simulink model "ex2_s"  (Simulink 7.9)
settings: Solver=ode45  StartTime=0.0  StopTime=10.0  RelTol=1e-3
undefined symbols (not defined in the file or in its folder): b1, den1, num1
settings Model: Creator=Theodor  LastModifiedBy=Theodor
settings DebuggingCC: SolverPrmCheckMsg=none

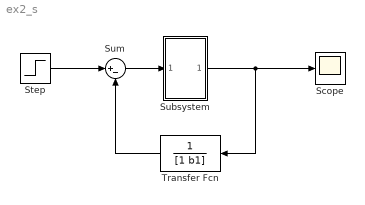
== system ex2_s ==
  Scope : Scope
  Step : Step  SampleTime=0
  Subsystem : Subsystem  mask{a=[3 6]}
      mask CallbackString:
      | if str2num(get_param(gcb,'a'))<0
      |     error('valoare negativa');
      | end
  Sum : Sum  Inputs=|+-
  Transfer Fcn : TransferFcn  Denominator=[1 b1]
  wires:
  Subsystem/1(Out1) -> Scope/1, Transfer Fcn/1
  Step/1 -> Sum/1
  Sum/1 -> Subsystem/1(In1)
  Transfer Fcn/1 -> Sum/2

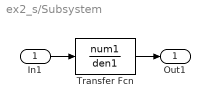
== system ex2_s/Subsystem ==
  In1 : Inport
  Transfer Fcn : TransferFcn  Numerator=num1  Denominator=den1
  Out1 : Outport
  wires:
  In1/1 -> Transfer Fcn/1
  Transfer Fcn/1 -> Out1/1
